simulink model "pruebaOPC"  (R2018a)
settings: Solver=VariableStepAuto  StartTime=0.0  StopTime=inf  RelTol=1e-3
libraries: simulink x4, opclib x3
settings Model: Creator=AndrewB  LastModifiedBy=AndrewB

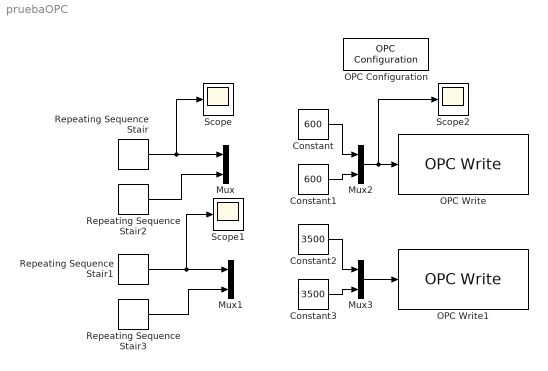
== system pruebaOPC ==
  Constant : Constant  Value=600
  Constant1 : Constant  Value=600
  Constant2 : Constant  Value=3500
  Constant3 : Constant  Value=3500
  Mux{,1..3} (4 alike) : Mux  Inputs=2
  OPC Configuration : opclib/OPC Configuration  opcServers=localhost/Kepware.KEPServerEX.V6/10  errMissingItems=Error  errReadWrite=Warn  errShutdown=Error  errRTViolation=Warn  rtEnable=on  speedup=1  showLatency=off  beingUsed=on
      settings: SourceProductName=OPC Toolbox  SourceProductBaseCode=OT
  OPC Write : opclib/OPC Write  serverHost=localhost  serverID=Kepware.KEPServerEX.V6  itemIDs=Bio_Channel.Bio.Group1.Pref, EnergAlter_Channel.EnergAlter.Group1.Pref  writeMode=Synchronous  updateRate=0
      settings: SourceProductName=OPC Toolbox  SourceProductBaseCode=OT
  OPC Write1 : opclib/OPC Write  serverHost=localhost  serverID=Kepware.KEPServerEX.V6  itemIDs=Bio_Channel.Bio.Group1.Qref, EnergAlter_Channel.EnergAlter.Group1.Qref  writeMode=Synchronous  updateRate=0
      settings: SourceProductName=OPC Toolbox  SourceProductBaseCode=OT
  Repeating Sequence Stair : simulink/Sources/Repeating Sequence Stair  OutValues=[0 134 500 200 100]'  tsamp=100  OutMin=[]  OutMax=[]  OutDataTypeStr=double  OutputDataTypeScalingMode=double  OutDataType=fixdt(0,8)  ConRadixGroup=Best Precision: Vector-wise  OutScaling=2^-12
  Repeating Sequence Stair1 : simulink/Sources/Repeating Sequence Stair  OutValues=[0 500 1500 3500 2000]'  tsamp=100  OutMin=[]  OutMax=[]  OutDataTypeStr=double  OutputDataTypeScalingMode=double  OutDataType=fixdt(0,8)  ConRadixGroup=Best Precision: Vector-wise  OutScaling=2^-12
  Repeating Sequence Stair2 : simulink/Sources/Repeating Sequence Stair  OutValues=[0 134 500 200 100]'  tsamp=100  OutMin=[]  OutMax=[]  OutDataTypeStr=double  OutputDataTypeScalingMode=double  OutDataType=fixdt(0,8)  ConRadixGroup=Best Precision: Vector-wise  OutScaling=2^-12
  Repeating Sequence Stair3 : simulink/Sources/Repeating Sequence Stair  OutValues=[0 134 500 200 100]'  tsamp=100  OutMin=[]  OutMax=[]  OutDataTypeStr=double  OutputDataTypeScalingMode=double  OutDataType=fixdt(0,8)  ConRadixGroup=Best Precision: Vector-wise  OutScaling=2^-12
  Scope : Scope
  Scope1 : Scope
  Scope2 : Scope
  wires:
  Repeating Sequence Stair/1 -> Mux/1, Scope/1
  Repeating Sequence Stair1/1 -> Mux1/1, Scope1/1
  Repeating Sequence Stair2/1 -> Mux/2
  Repeating Sequence Stair3/1 -> Mux1/2
  Mux2/1 -> Scope2/1, OPC Write/1
  Constant/1 -> Mux2/1
  Constant1/1 -> Mux2/2
  Constant3/1 -> Mux3/2
  Constant2/1 -> Mux3/1
  Mux3/1 -> OPC Write1/1
